simulink model "spped_control_bldc_3"  (R2024a)
settings: Solver=VariableStepAuto  StartTime=0.0  StopTime=10.0  RelTol=1e-3
libraries: simulink x12, spsMosfetLib x6, spsSeriesRLCBranchLib x2, spsDCVoltageSourceLib x1, slpidlib x1, spsPermanentMagnetSynchronousMachineLib x1, spsVoltageMeasurementLib x1, spspowerguiLib x1
settings Model: Creator=Abhi  LastModifiedBy=Abhi
settings SolverCC: AlgebraicLoopSolver=TrustRegion
settings DebuggingCC: UnconnectedInputMsg=warning  UnconnectedOutputMsg=warning  UnconnectedLineMsg=warning
settings ModelReferenceCC: EnableRefExpFcnMdlSchedulingChecks=on
settings RTWCC: GPUComputeCapability=3.5

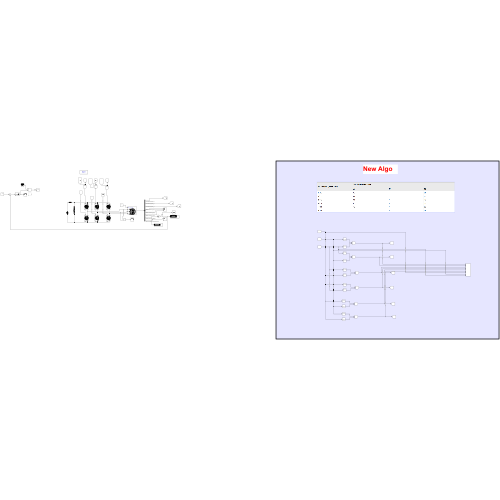
[thumbnail: Simulink's stored preview of the top-level diagram]
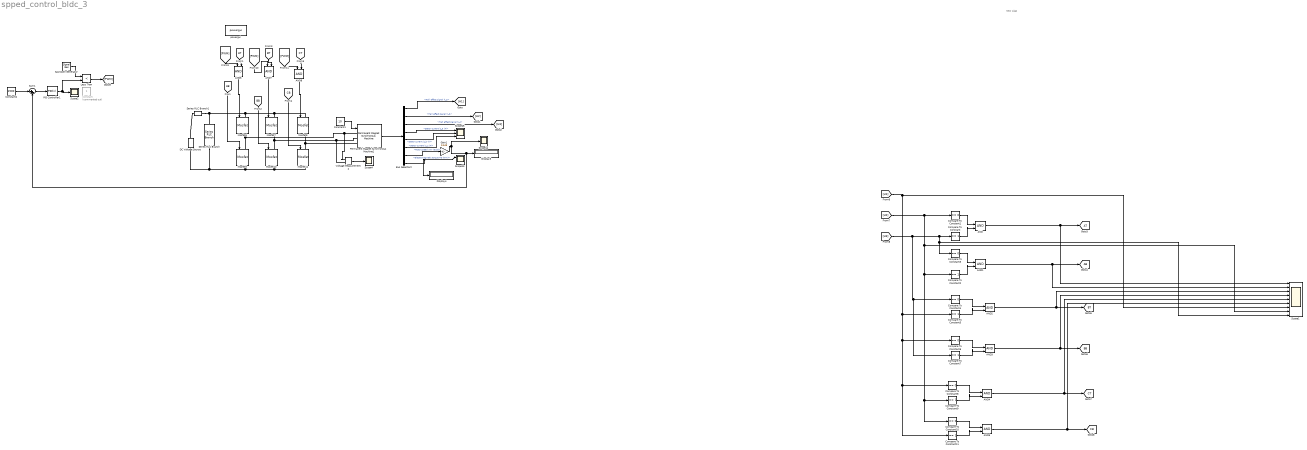
== system spped_control_bldc_3 ==
  note: New Algo
  AND{,1..8} (9 alike) : Logic  IconShape=distinctive  AllPortsSameDT=off  OutDataTypeStr=boolean
  Bus Selector2 : BusSelector  OutputSignals=Hall effect signal h_a,Hall effect signal h_b,Hall effect signal h_c,Stator current is_a (A),Stator current is_b (A),Stator current is_c (A),Rotor speed wm (rad/s),Electromagnetic torque Te (N*m)
  Compare To Constant{,2,5,7,9,11} (6 alike) : simulink/Logic and Bit Operations/Compare To Constant  relop===  const=1  OutDataTypeStr=boolean
  Compare To Constant{1,3..4,6,8,10} (6 alike) : simulink/Logic and Bit Operations/Compare To Constant  relop===  const=0  OutDataTypeStr=boolean
  Constant : Constant  Commented=on
  Constant1 : Constant  Value=10
  Constant2 : Constant  Value=1500
  DC Voltage Source : spsDCVoltageSourceLib/DC Voltage Source  Amplitude=200  Measurements=None
  Display3 : Display
  Display4 : Display
  Gain1 : Gain  Gain=9.549
  Less Than : RelationalOperator  Operator=<  OutDataTypeStr=boolean  RndMeth=Simplest  InputSameDT=off
  Mosfet{6..11} (6 alike) : spsMosfetLib/Mosfet  Ron=0.1  Lon=0  Rd=0.01  Vfd=0  IC=0  Rs=1e5  Cs=inf  Measurements=on
  PID Controller1 : slpidlib/PID Controller  Controller=PID  Form=Parallel  TimeDomain=Discrete-time  UseExternalTs=off  SampleTime=-1  IntegratorMethod=Forward Euler  FilterMethod=Forward Euler  ControllerParametersSource=internal  P=0.1  I=2  UseKiTs=off  D=0  UseExternalDerivativeSource=off  N=100  UseFilter=on  TunerSelectOption=Transfer Function Based (PID Tuner App)  InitialConditionSource=internal  InitialConditionForIntegrator=0  InitialConditionForFilter=0  DifferentiatorICPrevScaledInput=0  ExternalReset=none  TrackingMode=off  Kt=1  LimitOutput=on  SatLimitsSource=internal  UpperSaturationLimit=1  LowerSaturationLimit=-1  LinearizeAsGain=on  AntiWindupMode=none  Kb=1  LimitIntegrator=off  UpperIntegratorSaturationLimit=inf  LowerIntegratorSaturationLimit=-inf  POutMin=[]  POutMax=[]  IOutMin=[]  IOutMax=[]  DOutMin=[]  DOutMax=[]  NOutMin=[]  NOutMax=[]  SumOutMin=[]  SumOutMax=[]  SaturationOutMin=[]  SaturationOutMax=[]  PParamMin=[]  PParamMax=[]  IParamMin=[]  IParamMax=[]  DParamMin=[]  DParamMax=[]  NParamMin=[]  NParamMax=[]  KbParamMin=[]  KbParamMax=[]  KtParamMin=[]  KtParamMax=[]  KbOutMin=[]  KbOutMax=[]  KtOutMin=[]  KtOutMax=[]  IntegratorOutMin=[]  IntegratorOutMax=[]  FilterOutMin=[]  FilterOutMax=[]  SumI1OutMin=[]  SumI1OutMax=[]  SumI2OutMin=[]  SumI2OutMax=[]  SumI3OutMin=[]  SumI3OutMax=[]  SumI4OutMin=[]  SumI4OutMax=[]  SumDOutMin=[]  SumDOutMax=[]  DifferentiatorOutMin=[]  DifferentiatorOutMax=[]  FilterDiffOutCoefMin=[]  FilterDiffOutCoefMax=[]  ReciprocalOutMin=[]  ReciprocalOutMax=[]  SumDenOutMin=[]  SumDenOutMax=[]  SumNumOutMin=[]  SumNumOutMax=[]  DivideOutMin=[]  DivideOutMax=[]  UdiffTsProdOutMin=[]  UdiffTsProdOutMax=[]  NTsProdOutMin=[]  NTsProdOutMax=[]  UintegralTsProdOutMin=[]  UintegralTsProdOutMax=[]  UngainTsProdOutMin=[]  UngainTsProdOutMax=[]  ClampingZeroOutDataTypeStr=Inherit: Inherit via back propagation  ClampingZeroOutMin=[]  ClampingZeroOutMax=[]  FilterDenConstantOutDataTypeStr=Inherit: Inherit via back propagation  FilterDenConstantOutMin=[]  FilterDenConstantOutMax=[]  PCopyOutDataTypeStr=Inherit: Inherit via back propagation  PCopyOutMin=[]  PCopyOutMax=[]  NCopyOutDataTypeStr=Inherit: Inherit via back propagation  NCopyOutMin=[]  NCopyOutMax=[]  IntegratorContinuousStateAttributes=''  IntegratorStateMustResolveToSignalObject=off  IntegratorRTWStateStorageClass=Auto  FilterContinuousStateAttributes=''  FilterStateMustResolveToSignalObject=off  FilterRTWStateStorageClass=Auto  ParallelPVariant=InternalParameters  IdealPVariant=Disabled  IVariant=InternalParameters  DVariant=InternalParameters  IntegratorVariant=Discrete  SatVariant=Enabled  AWVariant=Passthrough  PCopyVariant=Disabled  TRVariant=Disabled  FdbkBlocksVariant=Forward  IdealPFdbkVariant=Disabled  SatFdbkVariant=Disabled  DerivativeFilterVariant=ForwardEulerFilter  NVariant=InternalParameters  NCopyVariant=Disabled  FilterICVariant=InternalICsFilter  IntegratorICVariant=InternalICs  ExternalResetVariant=Disabled  TRSumVariant=Passthrough  SumFdbkVariant=Disabled  SumVariant=Sum_PID  TsampFilterVariant=InternalTs  TsampNgainVariant=Passthrough  TsampIntegralVariant=Disabled_SignalSpec  ExternalSaturationOutDataTypeStr=Inherit: Same as second input  DerivativeSourceVariant=ErrorSignal
  Permanent Magnet Synchronous Machine1 : spsPermanentMagnetSynchronousMachineLib/Permanent Magnet Synchronous Machine  NbPhases=3  FluxDistribution=Trapezoidal  RotorType=Round  MechanicalLoad=Torque Tm  PresetModel="15:  87.75 Nm 560 Vdc 3000 RPM - 97.96 Nm"  ShowDetailedParameters=on  MeasurementBus=off  Resistance=0.05  Inductance=8.5e-3  dqInductances=[8.5e-3,8.5e-3]  La=0.000795  MachineConstant=Flux linkage established by magnets (V.s)  Flux=0.192  VoltageCst=160.8495  TorqueCst=1.536  Flat=120  Mechanical=[0.011 0.001417 4 0]  PolePairs=4  InitialConditions=[0,0, 0,0]  InitialConditions5ph=[0 0 0 0 0 0]  RefAngle=90 degrees behind phase A axis (modified Park)  IterativeDiscreteModel=Trapezoidal non iterative  TsBlock=-1  TsPowergui=0
  Sawtooth Generator : SignalGenerator  WaveForm=sawtooth  Frequency=10000
  Scope1 : Scope  NumInputPorts=9
  Scope13 : Scope  NumInputPorts=2
  Scope14 : Scope
  Scope15 : Scope  NumInputPorts=3
  Scope2 : Scope
  Scope4 : Scope
  Series RLC Branch : spsSeriesRLCBranchLib/Series RLC Branch  LConnTagsString=__new0  RConnTagsString=__new0  BranchType=C  Resistance=1  Inductance=1e-3  SetiL0=off  InitialCurrent=0  Capacitance=1e-3  Setx0=off  InitialVoltage=0  Measurements=None
  Series RLC Branch1 : spsSeriesRLCBranchLib/Series RLC Branch  LConnTagsString=__new0  RConnTagsString=__new0  BranchType=R  Resistance=3  Inductance=1e-3  SetiL0=off  InitialCurrent=0  Capacitance=1e-3  Setx0=off  InitialVoltage=0  Measurements=None
  Sum1 : Sum  Inputs=|+-
  Voltage Measurement2 : spsVoltageMeasurementLib/Voltage Measurement  PhasorSimulation=off  OutputType=Complex  PSBequivalent=0
  powergui : spspowerguiLib/powergui  Priority=1  SimulationMode=Discrete  SampleTime=1e-6  frequency=60  Iterations=50  frequencyindice=0  Pbase=100e6  ErrMax=1e-4  UnitsV=kV  UnitsW=MW  buscounter=0  FunctionMessages=off  echomessages=off  EnableUseOfTLC=off  CurrentSourceSwitches=off  DisableSnubberDevices=off  DisableRonSwitches=off  DisableVfSwitches=off  DisplayEquations=off  AutomaticDiscreteSolvers=off  SolverType=Tustin/Backward Euler (TBE)  Interpol=off  ExternalGateDelay=off  methode=off  Ts=100  x0status=blocks  SPID=on  SwTol=0  HookPort=off  NonlinearTolerance=0  nMaxIteration=15  ContinueOnMaxIteration=off  RestoreLinks=warning  ResistiveCurrentMeasurement=off  Frange=[0:2:500]  Ylog=off  Xlog=on  ShowGrid=off  save=off  variable=ZData  structure=0  ZoomFFT=off  StartTime=0.0  cycles=1  DisplayStyle=1  fundamental=60  FreqAxis=off  MaxFrequency=1000  frequencyindicesteady=1  RmsSteady=1  display=off
  tag scope: AB=global, AT=global, BB=global, BT=global, CB=global, CT=global
  wires:
  [H3] -> Compare To Constant7/1, Compare To Constant4/1, Compare To Constant3/1, Scope1/9, Compare To Constant/1
  Compare To Constant3/1 -> AND1/1
  [H1] -> Scope1/7, Compare To Constant11/1, Compare To Constant8/1, Compare To Constant6/1, Compare To Constant5/1
  Compare To Constant10/1 -> AND5/1
  AND4/1 -> [CT], Scope1/5
  AND3/1 -> [BB], Scope1/4
  Compare To Constant5/1 -> AND2/2
  Compare To Constant8/1 -> AND4/1
  Compare To Constant9/1 -> AND4/2
  AND/1 -> [AT], Scope1/1
  AND5/1 -> [CB], Scope1/6
  AND1/1 -> [AB], Scope1/2
  AND2/1 -> [BT], Scope1/3
  Compare To Constant2/1 -> AND1/2
  Compare To Constant6/1 -> AND3/1
  Compare To Constant7/1 -> AND3/2
  Compare To Constant4/1 -> AND2/1
  Compare To Constant/1 -> AND/2
  Compare To Constant11/1 -> AND5/2
  Compare To Constant1/1 -> AND/1
  [H2] -> Compare To Constant10/1, Compare To Constant9/1, Compare To Constant2/1, Scope1/8, Compare To Constant1/1
  Permanent Magnet Synchronous Machine1/1 -> Bus Selector2/1
  Bus Selector2/4 -> Scope15/1  "<Stator current is_a (A)>"
  Bus Selector2/8 -> Scope13/1, Display4/1  "<Electromagnetic torque Te (N*m)>"
  Voltage Measurement2/1 -> Scope4/1
  Gain1/1 -> Scope14/1, Sum1/2, Display3/1
  Bus Selector2/5 -> Scope15/2  "<Stator current is_b (A)>"
  Constant1/1 -> Permanent Magnet Synchronous Machine1/1
  Bus Selector2/7 -> Gain1/1  "<Rotor speed wm (rad/s)>"
  Bus Selector2/6 -> Scope15/3  "<Stator current is_c (A)>"
  Bus Selector2/1 -> [H1]  "<Hall effect signal h_a>"
  Bus Selector2/2 -> [H2]  "<Hall effect signal h_b>"
  Bus Selector2/3 -> [H3]  "<Hall effect signal h_c>"
  [AB] -> Mosfet9/1
  [BB] -> Mosfet10/1
  [CB] -> Mosfet11/1
  Sawtooth Generator/1 -> Less Than/1
  Less Than/1 -> [PWM]
  [AT] -> AND6/2
  [BT] -> AND7/2
  [CT] -> AND8/2
  AND6/1 -> Mosfet6/1
  AND7/1 -> Mosfet7/1
  AND8/1 -> Mosfet8/1
  [PWM] -> AND6/1
  [PWM] -> AND7/1
  [PWM] -> AND8/1
  PID Controller1/1 -> Less Than/2, Scope2/1
  Sum1/1 -> PID Controller1/1
  Constant2/1 -> Sum1/1
  connections:
  Mosfet9/RConn1 -- Series RLC Branch/RConn1 -- DC Voltage Source/LConn1 -- Mosfet10/RConn1 -- Mosfet11/RConn1
  Mosfet6/RConn1 -- Permanent Magnet Synchronous Machine1/LConn1 -- Voltage Measurement2/LConn1 -- Mosfet9/LConn1
  Mosfet8/LConn1 -- Series RLC Branch1/LConn1 -- Series RLC Branch/LConn1 -- Mosfet6/LConn1 -- Mosfet7/LConn1
  Mosfet8/RConn1 -- Permanent Magnet Synchronous Machine1/LConn3 -- Mosfet11/LConn1
  Voltage Measurement2/LConn2 -- Permanent Magnet Synchronous Machine1/LConn2 -- Mosfet7/RConn1 -- Mosfet10/LConn1
  DC Voltage Source/RConn1 -- Series RLC Branch1/RConn1
